simulink model "WEankle_controllerMaarten"  (R2018b)
settings: Solver=FixedStepDiscrete  StartTime=0.0  StopTime=inf  FixedStep=sampleTime  RelTol=1e-3
undefined symbols (not defined in the file or in its folder): DiscIntNeverNeededParam, forceplate, Joint_params, sampleTime
libraries: simulink x22, WE2_library x9, dspsigops x6, dspfdesign x3
(part 3 of 4)

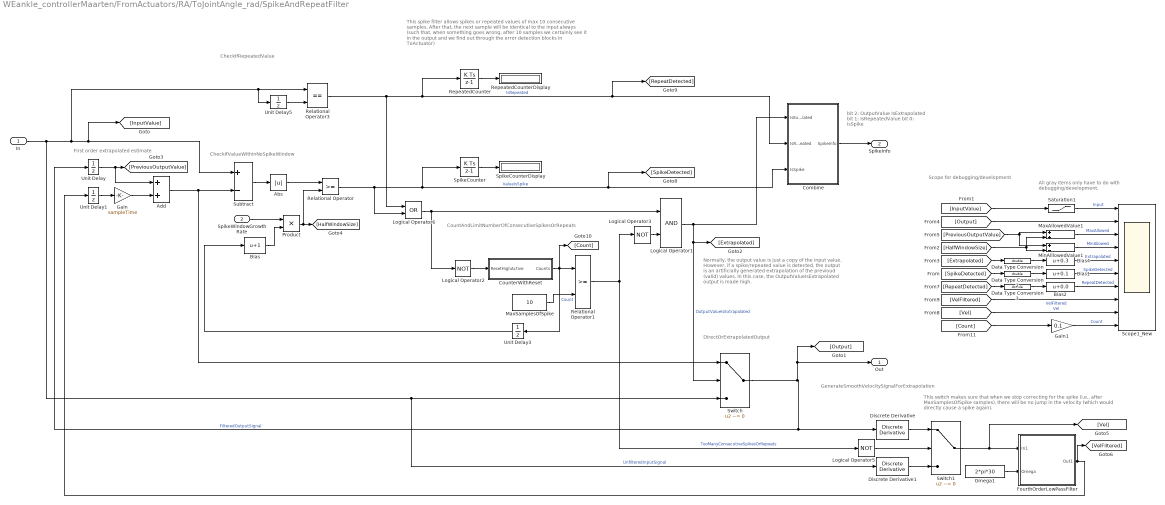
== system WEankle_controllerMaarten/FromActuators/RA/ToJointAngle_rad/SpikeAndRepeatFilter ==
  note: bit 2: OutputValue IsExtrapolated
      | bit 1: IsRepeatedValue
      | bit 0: IsSpike
  note: This switch makes sure that when we stop correcting for the spike (i.e., after MaxSamplesOfSpike samples), there will be no jump in the velocity (which would directly cause a spike again).
  note: This spike filter allows spikes or repeated values of max 10 consecutive samples. After that, the next sample will be identical to the input always (such that, when something goes wrong, after 10 samples we certainly see it in the output and we find out through the error detection blocks in ToActuator)
  note: First order extrapolated estimate
  note: CheckIfRepeatedValue
  note: CheckIfValueWithinNoSpikeWindow
  note: CountAndLimitNumberOfConsecutiveSpikesOrRepeats
  note: DirectOrExtrapolatedOutput
  note: GenerateSmoothVelocitySignalForExtrapolation
  note: All gray items only have to do with debugging/development.
  note: Scope for debugging/development
  note: Normally, the output value is just a copy of the input value. However, if a spike/repeated value is detected, the output is an artificially generated extrapolation of the previoud (valid) values. In this case, the OutputValueIsExtrapolated output is made high.
  In : Inport
  SpikeWindowGrowthRate : Inport  Port=2
  Abs : Abs
  Add : Sum
  Bias : Bias  Bias=1
  Bias1 : Bias  Bias=0.1
  Bias2 : Bias  Bias=0.0
  Bias4 : Bias  Bias=0.3
  Combine : Subsystem
  CounterWithReset : Subsystem
  Data Type Conversion : DataTypeConversion  OutDataTypeStr=double
  Data Type Conversion2 : DataTypeConversion  OutDataTypeStr=double
  Data Type Conversion3 : DataTypeConversion  OutDataTypeStr=double
  Discrete Derivative : simulink/Discrete/Discrete Derivative  gainval=1.0  ICPrevScaledInput=0.0  OutMin=[]  OutMax=[]  OutDataType=fixdt(1, 16)  OutScaling=2^-10  DoSatur=off
  Discrete Derivative1 : simulink/Discrete/Discrete Derivative  gainval=1.0  ICPrevScaledInput=0.0  OutMin=[]  OutMax=[]  OutDataType=fixdt(1, 16)  OutScaling=2^-10  DoSatur=off
  FourthOrderLowPassFilter : Subsystem
  Gain : Gain  Gain=sampleTime
  Gain1 : Gain  Gain=0.1
  Logical Operator1 : Logic  AllPortsSameDT=off  OutDataTypeStr=boolean
  Logical Operator2 : Logic  Operator=NOT  AllPortsSameDT=off  OutDataTypeStr=boolean
  Logical Operator3 : Logic  Operator=NOT  AllPortsSameDT=off  OutDataTypeStr=boolean
  Logical Operator5 : Logic  Operator=NOT  AllPortsSameDT=off  OutDataTypeStr=boolean
  Logical Operator6 : Logic  Operator=OR  AllPortsSameDT=off  OutDataTypeStr=boolean
  MaxAllowedValue1 : Sum
  MaxSamplesOfSpike : Constant  Value=10
  MinAlllowedValue1 : Sum  Inputs=+-
  Omega1 : Constant  Value=2*pi*30  OutDataTypeStr=double
  Product : Product
  Relational Operator : RelationalOperator  OutDataTypeStr=boolean  RndMeth=Nearest
  Relational Operator1 : RelationalOperator  OutDataTypeStr=boolean  RndMeth=Nearest
  Relational Operator3 : RelationalOperator  Operator===  OutDataTypeStr=boolean  RndMeth=Simplest
  RepeatedCounter : DiscreteIntegrator  SampleTime=-1  ICPrevOutput=DiscIntNeverNeededParam  ICPrevScaledInput=DiscIntNeverNeededParam
  RepeatedCounterDisplay : Display
  Saturation1 : Saturate  UpperLimit=6  LowerLimit=-6
  Scope1_New : Scope  NumInputPorts=10
  SpikeCounter : DiscreteIntegrator  SampleTime=-1  ICPrevOutput=DiscIntNeverNeededParam  ICPrevScaledInput=DiscIntNeverNeededParam
  SpikeCounterDisplay : Display
  Subtract : Sum  Inputs=+-
  Switch : Switch  Criteria=u2 ~= 0
  Switch1 : Switch  Criteria=u2 ~= 0
  Unit Delay{,1,3,5} (4 alike) : UnitDelay  SampleTime=sampleTime
  Out : Outport
  SpikeInfo : Outport  Port=2
  wires:
  Combine/1(SpikeInfo) -> SpikeInfo/1
  SpikeCounter/1 -> SpikeCounterDisplay/1
  RepeatedCounter/1 -> RepeatedCounterDisplay/1
  Logical Operator5/1 -> Switch1/2
  [Count] -> Gain1/1
  Gain1/1 -> Scope1_New/10  "Count"
  Relational Operator1/1 -> Logical Operator3/1, Logical Operator5/1  "TooManyConsecutiveSpikesOrRepeats"
  In/1 -> Discrete Derivative1/1, Switch/3, Unit Delay5/1, Relational Operator3/1, [InputValue], Subtract/1  "UnfilteredInputSignal"
  Unit Delay3/1 -> Bias/1
  Bias/1 -> Product/2
  SpikeWindowGrowthRate/1 -> Product/1
  Switch/1 -> [Output], Out/1, Unit Delay/1, Discrete Derivative/1  "FilteredOutputSignal"
  Add/1 -> Switch/1, Subtract/2
  Logical Operator1/1 -> Combine/1(IsExtrapolated), [Extrapolated], Switch/2  "OutputValueIsExtrapolated"
  Gain/1 -> Add/2
  Logical Operator6/1 -> Logical Operator1/1, Logical Operator2/1
  Unit Delay/1 -> [PreviousOutputValue], Add/1
  Abs/1 -> Relational Operator/1
  Subtract/1 -> Abs/1
  Product/1 -> Relational Operator/2, [HalfWindowSize]
  CounterWithReset/1(Counts) -> Relational Operator1/1, [Count], Unit Delay3/1  "Count"
  MaxSamplesOfSpike/1 -> Relational Operator1/2
  Discrete Derivative/1 -> Switch1/1
  Logical Operator3/1 -> Logical Operator1/2
  Discrete Derivative1/1 -> Switch1/3
  Unit Delay1/1 -> Gain/1
  Logical Operator2/1 -> CounterWithReset/1(ResetHighActive)
  Switch1/1 -> [Vel], FourthOrderLowPassFilter/1(In1)
  Omega1/1 -> FourthOrderLowPassFilter/2(Omega)
  FourthOrderLowPassFilter/1(Out1) -> [VelFiltered], Unit Delay1/1
  [Vel] -> Scope1_New/9  "Vel"
  Bias4/1 -> Scope1_New/5  "Extrapolated"
  Data Type Conversion2/1 -> Bias1/1
  [PreviousOutputValue] -> MaxAllowedValue1/1, MinAlllowedValue1/1
  [VelFiltered] -> Scope1_New/8  "VelFiltered"
  [Extrapolated] -> Data Type Conversion/1
  Data Type Conversion3/1 -> Bias2/1
  [InputValue] -> Saturation1/1
  Saturation1/1 -> Scope1_New/1  "Input"
  [SpikeDetected] -> Data Type Conversion2/1
  [Output] -> Scope1_New/2
  [RepeatDetected] -> Data Type Conversion3/1
  MaxAllowedValue1/1 -> Scope1_New/3  "MaxAllowed"
  MinAlllowedValue1/1 -> Scope1_New/4  "MinAllowed"
  [HalfWindowSize] -> MinAlllowedValue1/2, MaxAllowedValue1/2
  Data Type Conversion/1 -> Bias4/1
  Unit Delay5/1 -> Relational Operator3/2
  Relational Operator3/1 -> Logical Operator6/1, [RepeatDetected], Combine/2(IsRepeated), RepeatedCounter/1  "IsRepeated"
  Relational Operator/1 -> Logical Operator6/2, SpikeCounter/1, Combine/3(IsSpike), [SpikeDetected]  "ValueIsSpike"
  Bias2/1 -> Scope1_New/7  "RepeatDetected"
  Bias1/1 -> Scope1_New/6  "SpikeDetected"

== system WEankle_controllerMaarten/FromActuators/RA/ToJointAngle_rad/TakeDerivative ==
  note: DiscreteDerivativeOver2Samples
  note: We provide two ways of taking the derivative here:
      | dxdt = ( x(k)- x(k -1) ) / Ts
      | dxdt = ( x(k) - x(k -2) ) / (2*Ts)
      | The reason is that in TwinCAT we get a lot of jitter, which affects half of the samples. Therefore, comparing the current sample with two samples earlier may give more accurate results. this is, however, at a cost of latency.
  In1 : Inport
  Discrete Derivative : simulink/Discrete/Discrete Derivative  gainval=1.0  ICPrevScaledInput=0.0  OutMin=[]  OutMax=[]  OutDataType=fixdt(1, 16)  OutScaling=2^-10  DoSatur=off
  Manual Switch : ManualSwitch  CurrentSetting=0
  OneOverTwoSampleTime : Gain  Gain=1/(2*sampleTime)
  Subtract : Sum  Inputs=+-
  Unit Delay : UnitDelay  SampleTime=-1
  Unit Delay1 : UnitDelay  SampleTime=-1
  Out1 : Outport
  wires:
  Discrete Derivative/1 -> Manual Switch/1
  In1/1 -> Unit Delay/1, Subtract/1, Discrete Derivative/1
  Manual Switch/1 -> Out1/1
  Unit Delay/1 -> Unit Delay1/1
  Unit Delay1/1 -> Subtract/2
  Subtract/1 -> OneOverTwoSampleTime/1
  OneOverTwoSampleTime/1 -> Manual Switch/2

== system WEankle_controllerMaarten/Ankle Controller/COMverror and perturbation/TriggerPerturbation/Perturbation sync gait phase1/If Action Subsystem ==
  In1 : Inport
  Action Port : ActionPort  ActionType=then
  Out1 : Outport
  wires:
  In1/1 -> Out1/1

== system WEankle_controllerMaarten/Ankle Controller/COMverror and perturbation/TriggerPerturbation/Perturbation sync gait phase1/If Action Subsystem1 ==
  In1 : Inport
  Action Port : ActionPort  ActionType=then
  Out1 : Outport
  wires:
  In1/1 -> Out1/1

== system WEankle_controllerMaarten/FromActuators/RA/ToJointAngle_rad/SpikeAndRepeatFilter/Combine ==
  IsExtrapolated : Inport
  IsRepeated : Inport  Port=2
  IsSpike : Inport  Port=3
  Add : Sum  Inputs=+++
  Cast To Double : DataTypeConversion  OutDataTypeStr=double
  Cast To Double1 : DataTypeConversion  OutDataTypeStr=double
  Cast To Double2 : DataTypeConversion  OutDataTypeStr=double
  Gain : Gain  Gain=4
  Gain1 : Gain  Gain=2
  SpikeInfo : Outport
  wires:
  Cast To Double2/1 -> Add/3
  Cast To Double1/1 -> Gain1/1
  Cast To Double/1 -> Gain/1
  IsExtrapolated/1 -> Cast To Double/1
  IsRepeated/1 -> Cast To Double1/1
  Add/1 -> SpikeInfo/1
  Gain1/1 -> Add/2
  Gain/1 -> Add/1
  IsSpike/1 -> Cast To Double2/1

== system WEankle_controllerMaarten/FromActuators/RA/ToJointAngle_rad/SpikeAndRepeatFilter/CounterWithReset ==
  note: Stopwatch -
      | Outputs time in seconds.
      | Reset during high level of Rest pulse
  ResetHighActive : Inport
  Counter Free-Running : simulink/Sources/Counter Free-Running  NumBits=32  tsamp=-1
  Data Type Conversion : DataTypeConversion  OutDataTypeStr=double
  Latch : Subsystem
  Subtract : Sum  Inputs=+-
  Counts : Outport
  wires:
  Counter Free-Running/1 -> Latch/1(In1), Subtract/1
  Subtract/1 -> Data Type Conversion/1
  Latch/1(Out1) -> Subtract/2  "startTime"
  Data Type Conversion/1 -> Counts/1
  ResetHighActive/1 -> Latch/Enable

== system WEankle_controllerMaarten/FromActuators/RA/ToJointAngle_rad/SpikeAndRepeatFilter/FourthOrderLowPassFilter ==
  In1 : Inport
  Omega : Inport  Port=2
  Filter1 : MATLAB Function  TreatAsAtomicUnit=on  mask{sampleTime=sampleTime}
      mask prompts: sampleTime "Sample Time"
  Filter2 : MATLAB Function  TreatAsAtomicUnit=on  mask{sampleTime=sampleTime}
      mask prompts: sampleTime "Sample Time"
  Out1 : Outport
  wires:
  Omega/1 -> Filter1/2(OmegaFilter), Filter2/2(OmegaFilter)
  Filter2/1(y) -> Out1/1
  Filter1/1(y) -> Filter2/1(x)
  In1/1 -> Filter1/1(x)

== system WEankle_controllerMaarten/FromActuators/RA/ToJointAngle_rad/SpikeAndRepeatFilter/CounterWithReset/Latch ==
  In1 : Inport
  Enable : EnablePort
  Out1 : Outport
  wires:
  In1/1 -> Out1/1

== matlab function WEankle_controllerMaarten/Ankle Controller/Eventdetection/StrideTimeEstimator/MATLAB Function ==
  data: fLeftCross input; fLeftThresh input; phase_left output; fRightCross input; fRightThresh input; time input; phase_right output
function [phase_left, phase_right] = fcn(fLeftCross, fLeftThresh, fRightCross, fRightThresh, time)

persistent time_heel2heel_right
persistent time_heellast_right
persistent tdm_right
persistent time_heel2heel_left
persistent time_heellast_left
persistent tdm_left

if(isempty(time_heel2heel_left))
   time_heel2heel_right = zeros(4,1);
   time_heellast_right = -1e5;
   tdm_right = 0.1;
   
   time_heel2heel_left = zeros(4,1);
   time_heellast_left = -1e5;
   tdm_left = 0.1;
end
%% left
phase_left = (time - time_heellast_left)/(tdm_left+eps)*100;
if(fLeftCross~=0||(phase_left>100&&fLeftThresh==1))
    td_new  = time - time_heellast_left;
    if((td_new>0.8*tdm_left)||any(time_heel2heel_left>10))
        time_heellast_left = time;
        time_heel2heel_left(2:end) = time_heel2heel_left(1:end-1);
        time_heel2heel_left(1) = td_new;
        tdm_left = mean(time_heel2heel_left);
    end
end


%% right
phase_right = (time - time_heellast_right)/(tdm_right+eps)*100;
if(fRightCross~=0||(phase_right>100&&fRightThresh==1))
    td_new  = time - time_heellast_right;
    if((td_new>0.8*tdm_right)||any(time_heel2heel_right>10))
        time_heellast_right = time;
        time_heel2heel_right(2:end) = time_heel2heel_right(1:end-1);
        time_heel2heel_right(1) = td_new;
        tdm_right = mean(time_heel2heel_right);
    end
end

== matlab function WEankle_controllerMaarten/Ankle Controller/Eventdetection/COP detection (treadmill)/MATLAB Function1 ==
  data: x input; y output; OmegaFilter input; sampleTime input
function y = Filter2ndOrder(x, OmegaFilter, sampleTime)
%#codegen

persistent yd_prev y_prev;
if isempty(yd_prev)
    yd_prev = zeros(6,1); 
    y_prev = zeros(6,1);  %Derivative of the above signal
end

% Do 2nd order filtering with given omega and zeta=0.7; input of filter
% is vel_inc_sampleTime_unfilt; output is y (we assign to vel_inc_s
% later). 
if OmegaFilter==0 || isinf(OmegaFilter)
    y = x;
    y_prev = y;
    yd_prev = zeros(6,1); 
else
    zeta = 0.7;
    ydd = OmegaFilter^2 * (x - y_prev) - 2*zeta*OmegaFilter* yd_prev;
    yd = yd_prev + ydd * sampleTime;
    y = y_prev + yd * sampleTime;

    y_prev = y; yd_prev = yd;
end

== matlab function WEankle_controllerMaarten/Ankle Controller/MATLAB Function5 ==
  data: e0 input; G input; SolGains output; COMd input
function SolGains  = CombineSoleusGains(e0,G,COMd)
% input arguments:

SolGains = [e0; G; COMd];

== matlab function WEankle_controllerMaarten/ForcePlate/Calibration/MATLAB Function ==
  data: left input; left_calib output; right input; start input; right_calib output; caltime_s input
function [left_calib, right_calib] = calibrateOffset(left, right, start, caltime_s)
persistent calibrated
persistent offcum_left
persistent offcum_right
persistent counter
persistent nosamp

if(isempty(calibrated))
   calibrated = false;
   offcum_left = left*0;
   offcum_right = right*0;
   counter = 0;
   nosamp = max(1, floor(caltime_s*1000));
end

if(start == 1)
    counter = 0;
    calibrated = false;
    offcum_left = left*0;
    offcum_right = right*0;
    nosamp = max(1, floor(caltime_s*1000));
end

if(calibrated)
    left_calib = left - offcum_left;
    right_calib = right - offcum_right;
else
    if(~calibrated)
        counter = counter + 1;
        offcum_left = offcum_left + left/(nosamp);
        offcum_right = offcum_right + right/(nosamp);
        if(counter >= nosamp)
            calibrated = true;
        end
    end
    left_calib = left;
    right_calib = right;
end

== matlab function WEankle_controllerMaarten/Ankle Controller/Eventdetection/COP detection (treadmill)/MATLAB Function2 ==
  data: x input; y output; OmegaFilter input; sampleTime input
function y = Filter2ndOrder(x, OmegaFilter, sampleTime)
%#codegen

persistent yd_prev y_prev;
if isempty(yd_prev)
    yd_prev = zeros(6,1); 
    y_prev = zeros(6,1);  %Derivative of the above signal
end

% Do 2nd order filtering with given omega and zeta=0.7; input of filter
% is vel_inc_sampleTime_unfilt; output is y (we assign to vel_inc_s
% later). 
if OmegaFilter==0 || isinf(OmegaFilter)
    y = x;
    y_prev = y;
    yd_prev = zeros(6,1); 
else
    zeta = 0.7;
    ydd = OmegaFilter^2 * (x - y_prev) - 2*zeta*OmegaFilter* yd_prev;
    yd = yd_prev + ydd * sampleTime;
    y = y_prev + yd * sampleTime;

    y_prev = y; yd_prev = yd;
end

== matlab function WEankle_controllerMaarten/Ankle Controller/COMverror and perturbation/TriggerPerturbation/Perturbation sync gait phase1/TimeBetweenPert ==
  data: TimeBetweenPert input; timesvector input; Allow output; Delivered input
function Allow = fcn(TimeBetweenPert,timesvector,Delivered)
% To randomize the time between perturbations (min 6s)
persistent i 
persistent TimeSelector 
persistent flagfirst %flag to indicate first time
if isempty(i)
    i = 1;
    flagfirst = 1;
end
if Delivered == 1 && ~flagfirst %Perturbation delivered. Go to next element of timesVector avoiding a false entrance the first time
    i = i+1;
end
%% Assign new time
len = length(timesvector);
if i > len %reset the index when all perturbations from the vector are done
    i = 1;
end
TimeSelector = timesvector(i);

if TimeSelector < 6
    TimeSelector = 6;
end
%% Allow new perturbation or not
if TimeBetweenPert >= TimeSelector
    Allow = 1;
else
    Allow = 0;
end
%%
flagfirst = 0;

== matlab function WEankle_controllerMaarten/Ankle Controller/Eventdetection/Subsystem/MATLAB Function ==
  data: f input; y output; nf input; nf_1 input; th input
function y = fcn(f,nf,nf_1,th)

maxCounter = 200; %time to wait in zero
persistent counter
persistent out
if isempty(counter)
    counter = maxCounter+1;
    out = f;
end

if (nf == 0) && (nf_1 < -50)
    out = 0;
    counter = 0;
else
    counter = counter+1;
    if counter > maxCounter
        if (f > -th) && (f < th) && (nf == 0)
            out = 0;
        else
            out = f;
        end
    end
end

y = out;

== matlab function WEankle_controllerMaarten/Ankle Controller/Eventdetection/StrideTimeEstimator/MATLAB Function3 ==
  data: fLeftCross input; fLeftThresh input; phase_left output; fRightCross input; fRightThresh input; time input; phase_right output; SingleL input; SingleR input; reset input
function [phase_left, phase_right] = fcn(fLeftCross, fLeftThresh, fRightCross, fRightThresh, time, SingleL, SingleR, reset)

persistent time_heel2heel_right
persistent time_heellast_right
persistent tdm_right
persistent time_heel2heel_left
persistent time_heellast_left
persistent tdm_left
persistent  phase_left2
persistent  phase_right2

if(isempty(time_heel2heel_left) || reset==1)
   time_heel2heel_right = zeros(4,1);
   time_heellast_right = -1e5;
   tdm_right = 0.1;
   
   time_heel2heel_left = zeros(4,1);
   time_heellast_left = -1e5;
   tdm_left = 0.1;
   
    phase_left2 = 0; %Used to reset the left phase when prepositioning of left leg is detected (SingleL 1 to 0)
    phase_right2 = 0; %Used to reset the right phase when prepositioning of right leg is detected (SingleR 1 to 0)
end
%% left
phase_left = (time - time_heellast_left)/(tdm_left+eps)*100 - phase_left2;
% if(fLeftCross~=0||(phase_left>100&&fLeftThresh==1))

if(SingleR)
    phase_left2 = phase_left;
end
if((fLeftCross~=0||(phase_left>100&&fLeftThresh==1)))
    td_new  = time - time_heellast_left;
    phase_left2 = 0;
    if((td_new>0.8*tdm_left)||any(time_heel2heel_left>10))
        time_heellast_left = time;
        time_heel2heel_left(2:end) = time_heel2heel_left(1:end-1);
        time_heel2heel_left(1) = td_new;
        tdm_left = mean(time_heel2heel_left);
    end
end


%% right
phase_right = (time - time_heellast_right)/(tdm_right+eps)*100 - phase_right2;
% if(fRightCross~=0||(phase_right>100&&fRightThresh==1))
if(SingleL)
    phase_right2 = phase_right;
end
if(fRightCross~=0||(phase_right>100&&fRightThresh==1))
    td_new  = time - time_heellast_right;
    phase_right2 = 0;
    if((td_new>0.8*tdm_right)||any(time_heel2heel_right>10))
        time_heellast_right = time;
        time_heel2heel_right(2:end) = time_heel2heel_right(1:end-1);
        time_heel2heel_right(1) = td_new;
        tdm_right = mean(time_heel2heel_right);
    end
end

== matlab function WEankle_controllerMaarten/FromActuators/RA/CheckOperationEnabled ==
  data: u input; y output
function y = fcn(u)
%#codegen
% Extract the 'Operation Enabled' bit from the Status Word
y = double(bitget(u, 2+1)); % bitget is one-based

== matlab function WEankle_controllerMaarten/FromActuators/RA/ToJointAngle_rad/FilterFourthOrder/Filter1 ==
  data: x input; OmegaFilter input; y output; sampleTime parameter
function y = Filter2ndOrder(x, OmegaFilter, sampleTime)
%#codegen

persistent yd_prev y_prev;
if isempty(yd_prev)
    yd_prev = 0; 
    y_prev = 0; %Derivative of the above signal
end;

% Do 2nd order filtering with given omega and zeta=0.7; input of filter
% is vel_inc_sampleTime_unfilt; output is y (we assign to vel_inc_s
% later). 
if OmegaFilter==0 || isinf(OmegaFilter)
    y=x;
    y_prev=y;
    yd_prev =0;
else
    zeta = 0.7;
    ydd = OmegaFilter^2 * (x - y_prev) - 2*zeta*OmegaFilter* yd_prev;
    yd = yd_prev + ydd * sampleTime;
    y = y_prev + yd * sampleTime;

    y_prev = y; yd_prev = yd;
end;

== matlab function WEankle_controllerMaarten/Ankle Controller/Eventdetection/Heels movement/MATLAB Function2 ==
  data: gainL output; COPyL input; gainR output; COPyR input
function [gainL,gainR] = Stance(COPyL,COPyR)
%#codegen
if COPyR == 0
    gainR = 0;
else
    gainR = 1;
end

if COPyL == 0
    gainL = 0;
else
    gainL = 1;
end

end

== matlab function WEankle_controllerMaarten/Ankle Controller/COMverror and perturbation/TriggerPerturbation/PushOrPull ==
  data: Perturb input; vectorPushPull input; NewPert output; Delivered input
function NewPert = fcn(Perturb,vectorPushPull,Delivered)
% To randomize pushes and pulls
persistent i 
persistent Selector 
persistent flagfirst %flag to indicate first time
if isempty(i)
    i = 1;
    flagfirst = 1;
end
if Delivered == 1 && ~flagfirst %Perturbation delivered. Go to next element of timesVector avoiding a false entrance the first time
    i = i+1;
end
%%
len = length(vectorPushPull);
if i > len %reset the index when all perturbations from the vector are done
    i = 1;
end
Selector = vectorPushPull(i);

if Selector < -1
    Selector = -1;
elseif Selector > 1
    Selector = 1;
end
%% 
NewPert = Selector*Perturb;
%%
flagfirst = 0;

== matlab function WEankle_controllerMaarten/Ankle Controller/COMverror and perturbation/COMvError/MATLAB Function1 ==
  data: ShutDown input; PertDetect input; TriggerPush output
function TriggerPush = fcn(ShutDown,PertDetect)
if ShutDown == 0
    TriggerPush = PertDetect;
else
    TriggerPush = 0;
end

== matlab function WEankle_controllerMaarten/Ankle Controller/COMverror and perturbation/COMvError/Signal learner/MATLAB Function ==
  data: reset input; t input; trigger input; signal input; signal_learned output; n_strides_ output; n_ output; m_ output; output_duration_ output; n_rep input; perturbation output; threshPert input; DataLost input; ShutDown output
function [signal_learned,n_strides_,n_,m_,output_duration_,perturbation,ShutDown] = signal_learner(reset,t,trigger,signal,n_rep,threshPert,DataLost)
%     n_rep = how many signals period will be averaged
n_storage = 2000; %stored signal will be 2000 elements long. playback will be interpolated
n_buffer_size = 4000; %can maximally read 4000;
perturbation = 0;
ShutDown = 0; %No trigger the controller if DataLost or if we are in the first n_rep strides
persistent n %elements of vector
persistent n_strides % total number of strides
persistent m %Pointer for recording each stride in buffer (1:n_rep)
persistent t0 % moment in time of last stride
persistent last_buffer
persistent output_signal_buffer
persistent output_signal
persistent output_duration
persistent output_duration_buffer
persistent maximums
persistent MaxAver

if isempty(n)
    n = 1;
    m = 1;
    t0 = 0;
    last_buffer = zeros(1,n_buffer_size);
    output_signal_buffer = zeros(n_rep,n_storage);
    output_signal = zeros(1,n_storage);
    output_duration_buffer = zeros(n_rep,1);
    n_strides = 0;
    output_duration = 1;
    % Added Cristina
    maximums = 200*ones(n_rep,1); %to store the maximums of previous steps
    MaxAver = 200; % This number multiplied by 1.5 is the one above which a perturbation is supposed to happen,
    %     and thereby, that step will be excluded to calculate the mean
end
if ~DataLost && ~reset
    t_rel = t-t0;
    if (trigger && t_rel > 0.1) %if trigger happens, note down the absolute time when that was
        n_strides = n_strides+1; %counting number of strides
        last_stride_duration = t-t0;
        
        t0 = t; %Reset the moment when the last stride happened
        %% Added Cristina
        % See if there was a perturbation in the last step
        Perturbation = 0; % Init perturbation in the last step
        leng = length(last_buffer(1:min([n,n_buffer_size])));
        for i = 1:leng
            element = last_buffer(i);
            if element > 1.5*MaxAver % A perturbation was detected in the last step
                Perturbation = 1;
            end
        end
        
        %% Changed Cristina
        if n_strides >= 3
            if (last_stride_duration > 0.5*output_duration)% to avoid false triggers
                enter = 1;
            else
                enter = 0;
            end
        else
            enter = 1;
        end
        if (last_stride_duration > 0) && enter % otherwise failure at start or false trigger  
            % If there was no perturbation, take that step into account.
            % Otherwise, exclude it
            if ~Perturbation %in the last step
                %interpolate regardless of last duration to n_storage elements
%                 if n == 1
%                     n = n+1;
%                 end
                output_signal_buffer(m,:) = ...
                    interp1(...
                    linspace(0,last_stride_duration,n),... %vector of n elements
                    last_buffer(1:min([n,n_buffer_size])),... %only read up to incl. n elements, if bigger than n_buffer size, then we need to limit.
                    linspace(0,last_stride_duration,n_storage)); %remap that to a new 'x' with n_storage elements
                output_signal = mean(output_signal_buffer); %averages over n_rep stored signals
                
                output_duration_buffer(m) = last_stride_duration;
                output_duration = mean(output_duration_buffer); %duration is average of last n_rep times
                
                maximums(m) = max(last_buffer(1:min([n,n_buffer_size]))); %store the new maximum of current step
                MaxAver = mean(maximums); %calculate the average of maximums found in the last n_rep
                
                m = m+1;
                if m > n_rep
                    m = 1;
                end
            end
            if (n_strides <= n_rep)
                output_duration = last_stride_duration;
            end
            %last_buffer = zeros() %is not required due to 1:n
            n = 1;
        end
    end
end
if ~DataLost && ~reset
    %% process input
    t_rel = t-t0;
    last_buffer(min([n n_buffer_size])) = signal;
    
    %% generate output
    fractional_index = t_rel/output_duration * (n_storage-1);
    rounded_index = min([1+floor(fractional_index),n_storage]); %cannot overflow
    fraction = 1+fractional_index - rounded_index;
    
    %linearly interpolate
    if (rounded_index >= n_storage - 1)
        signal_learned = output_signal(n_storage-1);
    else
        signal_learned = output_signal(rounded_index)*(1-fraction) + output_signal(rounded_index+1)*fraction;
    end
    
    %debug output
    n_strides_ = n_strides;
    n_ = n;
    m_ = m;
    output_duration_ = output_duration;
    if signal > threshPert*MaxAver
        perturbation = 1;
    end
else
    %debug output
    n_strides_ = n_strides;
    n_ = n;
    m_ = m;
    output_duration_ = output_duration;
    perturbation = 0;
    signal_learned = 0;
end

%do not output anything learned in first n_rep strides.
if (n_strides <= n_rep) || DataLost || reset
    signal_learned = 0;
    output_duration_ = 0;%last_stride_duration;
    ShutDown = 1;
end
if ~DataLost && ~reset
    %shift signal storage pointer, avoid overflow
    n = n+1;
else
    n = 1;
end
end

== matlab function WEankle_controllerMaarten/Ankle Controller/COMverror and perturbation/COMvError/Data lost detection/MATLAB Function1 ==
  data: u input; y output; u_1 input
function y = fcn(u,u_1)
% input signal u = xVelCOM
% output y = data lost detection (1 or 0)
y = 0;
if u == u_1 % The new data is equal to the previous one --> See how Qualisys will send it since NaN is not supported
    y = 1; % Data lost
else
    y = 0; % Data good
end

== matlab function WEankle_controllerMaarten/Ankle Controller/COMverror and perturbation/COMvError/Data lost detection/MATLAB Function2 ==
  data: DataLost input; DataLost_1 input; ErrorOut output; ErrorIn input; avoid output
function [ErrorOut,avoid] = fcn(DataLost,DataLost_1,ErrorIn)
% ErrorOut is the new error corrected when data lost

maxCounter = 1500; %time to wait after a DataLost detection to let the controller works again (1.5s)
persistent counter
if isempty(counter)
    counter = maxCounter+1;
end

ErrorOut = ErrorIn;
avoid = 0;

if DataLost == 1 % Data lost
    ErrorOut = 0; 
    avoid = 1;
elseif DataLost == 0 && DataLost_1 == 1 % Data just recovered after a loss
    counter = 1;
    ErrorOut = 0; 
    avoid = 1;
elseif DataLost == 0 && DataLost_1 ~= 1 % Good data
    if counter <= maxCounter % Wait 1.5s after data has been recovered to generate the newError
        ErrorOut = 0;
        avoid = 1;
        counter = counter + 1;
    else
        ErrorOut = ErrorIn;
        avoid = 0;
    end
end

== matlab function WEankle_controllerMaarten/Ankle Controller/COMverror and perturbation/COMvError/PerturbationDetectionFromError ==
  data: t input; trigger input; signal input; n_rep input; push output; maxAver output; rangeAver output; threshPert input; DataLost input
function [push,maxAver,rangeAver] = PerturbationDetectionFromError(t,trigger,signal,n_rep,threshPert,DataLost)
    n_buffer_size = 4000; %can maximally read 4000;
    push = 0; 
    
    persistent n %elements of vector
    persistent n_strides % total number of strides
    persistent m %Pointer for recording each stride in buffer (1:n_rep)
    persistent t0 % moment in time of last stride
    persistent last_buffer
    persistent maximums
    persistent MaxAver
    persistent minimums
    persistent MinAver
    persistent RangeAver

    if isempty(n)
       n = 1;
       m = 1;
       t0 = 0;
       last_buffer = zeros(1,n_buffer_size);
       n_strides = 0;

       maximums = 50*ones(n_rep,1); %to store the maximums of previous steps
       MaxAver = 50; % This number multiply by 1.5 is the one above which a push perturbation is supposed to happen,
%     and thereby, that step will be excluded to calculate the mean of
%     maximums
       minimums =  -120*ones(n_rep,1);
       MinAver = -120;
       RangeAver = 170;
    end
if ~DataLost
    t_rel = t-t0;
    if (trigger && t_rel > 0.1) %if trigger happens, note down the absolute time when that was
        n_strides = n_strides+1; %counting number of strides
        last_stride_duration = t-t0;

        t0 = t; %Reset the moment when the last stride happened
        %% Added Cristina
        % See if there was a perturbation in the last step
        Push = 0; % Init perturbation in the last step
        leng = length(last_buffer(1:min([n,n_buffer_size])));
        for i = 1:leng
            element = last_buffer(i);
            if element > 1.5*MaxAver % A perturbation was detected in the last step
                Push = 1;
            end
        end
        
        %% Changed Cristina
        if (last_stride_duration > 0) %otherwise failure at start
            % If there was no perturbation, take that step into account.
            % Otherwise, exclude it
            if ~Push %in the last step                
                maximums(m) = max(last_buffer(1:min([n,n_buffer_size]))); %store the new maximum of current step
                MaxAver = mean(maximums); %calculate the average of maximums found in the last n_rep
                
                minimums(m) = min(last_buffer(1:min([n,n_buffer_size]))); %store the new minimum of current step
                MinAver = mean(minimums); %calculate the average of minimums found in the last n_rep
                RangeAver = MaxAver - MinAver;
                
                m = m+1;
                if m > n_rep 
                    m = 1;
                end
            end

            n = 1;
        end
    end
end
if ~DataLost
    %% process new data
    last_buffer(min([n n_buffer_size])) = signal;
    
    %% generate output
    if signal > threshPert*RangeAver 
        push = 1;
    end
    maxAver = MaxAver;
    rangeAver = RangeAver;
    
else
    maxAver = MaxAver;
    rangeAver = RangeAver;
    push = 0;
end
%do not output anything learned in first n_rep strides.
if (n_strides <= n_rep) || DataLost
    push = 0;
end

if ~DataLost
    %shift signal storage pointer, avoid overflow
    n = n+1;
else
    n = 1;
end
end

== matlab function WEankle_controllerMaarten/Ankle Controller/COMverror and perturbation/COMvError/PertDetection/MATLAB Function1 ==
  data: PertFromError input; PertDetect output; PertFromInput input; avoid input; StartPertFromError input
function PertDetect = NotTriggerIfDataLost(PertFromError,PertFromInput,avoid,StartPertFromError)
% PertFromError is already including the data lost because the error will
% be zero if that happens. But it could be that PertFromInput says there is
% a perturbation, and that is why this is needed

%avoid because data lost

persistent CounterPertError
if isempty(CounterPertError)
    CounterPertError = 0;
end
if StartPertFromError
    CounterPertError = CounterPertError +1;
end
%Discard the first two perturbations detected from error
if (PertFromError || PertFromInput) && ~avoid && (CounterPertError > 2)  %Detect a new perturbation
    PertDetect = 1;
else
    PertDetect = 0;
end

== matlab function WEankle_controllerMaarten/Ankle Controller/COMverror and perturbation/COMvError/PertDetection/MATLAB Function2 ==
  data: Pert input; PertDetect output; Pert_1 input
function PertDetect = WaitForNewDetect(Pert,Pert_1)
PertDetect = 0;
% Wait 2s to trigger a new perturbation if a previous one was detected

maxCounter = 2000; %time to wait after a Perturbation detection to detect a new one
persistent counter
if isempty(counter)
    counter = maxCounter+1;
end

if Pert_1 == 0 && Pert == 1 %New possible perturbation
    if counter > maxCounter
        PertDetect = Pert;
    else
        PertDetect = 0;
    end
elseif Pert_1 == 1 && Pert == 1 %middle of a perturbation
    if counter > maxCounter
        PertDetect = Pert;
    else
        PertDetect = 0;
    end
elseif Pert_1 == 1 && Pert == 0 % end of a perturbation
    counter = 1;
    PertDetect = Pert;
end

counter = counter + 1;

== matlab function WEankle_controllerMaarten/Ankle Controller/Eventdetection/Subsystem1/MATLAB Function ==
  data: f input; y output; nf input; nf_1 input; th input
function y = fcn(f,nf,nf_1,th)

maxCounter = 200; %time to wait in zero
persistent counter
persistent out
if isempty(counter)
    counter = maxCounter+1;
    out = f;
end

if (nf == 0) && (nf_1 < -50)
    out = 0;
    counter = 0;
else
    counter = counter+1;
    if counter > maxCounter
        if (f > -th) && (f < th) && (nf == 0)
            out = 0;
        else
            out = f;
        end
    end
end

y = out;

== matlab function WEankle_controllerMaarten/Ankle Controller/Eventdetection/MATLAB Function2 ==
  data: COPyL input; leftFront output; COPyR input; rightFront output; singleLeft output; singleRight output; COPyL_1 input; COPyR_1 input
% function [LeftFront,RightFront,SingleLeft,SingleRight] = DetectionFrontFoot(COPyL,COPyR,COPyL_1,COPyR_1)
function [leftFront,rightFront,singleLeft,singleRight] = DetectionFrontFoot(COPyL,COPyR,COPyL_1,COPyR_1)
%#codegen
% LeftFront = 0; 
% RightFront = 0;
% SingleRight = 0;
% SingleLeft = 0;

persistent LeftFront
persistent RightFront
persistent SingleRight
persistent SingleLeft

maxCounter = 3; %time to wait to avoid false detection
maxCounterStance = 4;
persistent counter
persistent counterStance
if isempty(counter)
    counter = maxCounter+1;
    counterStance = maxCounterStance+1;
    LeftFront = 0;
    RightFront = 0;
    SingleRight = 0;
    SingleLeft = 0;
end

%%
if (COPyL~=0) && (COPyR~=0) && ((COPyL_1 == 0) || (COPyR_1 == 0)) %Possible init of double stance
    counterStance = 0;
elseif (COPyL~=0) && (COPyR~=0) && (COPyL_1 ~= 0) && (COPyR_1 ~= 0) % Possible double stance
    counterStance = counterStance + 1;
    if counterStance > maxCounterStance
        if COPyL > COPyR %Left in front
            LeftFront = 1;
            RightFront = 0;
            SingleRight = 0;
            SingleLeft = 0;
        elseif COPyL < COPyR %Rigth in front
            LeftFront = 0;
            RightFront = 1;
            SingleRight = 0;
            SingleLeft = 0;
        end
    end
    
% if (COPyL~=0) && (COPyR~=0) %Double stance
%     if COPyL > COPyR %Left in front
%         LeftFront = 1;
%         RightFront = 0;
%         SingleRight = 0;
%         SingleLeft = 0;
%     elseif COPyL < COPyR %Rigth in front
%         LeftFront = 0;
%         RightFront = 1;
%         SingleRight = 0;
%         SingleLeft = 0;
%     end
elseif (COPyL == 0) && (COPyR == 0) %No one on the treadmill
    LeftFront = 0;
    RightFront = 0;
    SingleRight = 0;
    SingleLeft = 0;
elseif (COPyL == 0) && (COPyL_1 ~= 0) && (COPyR ~= 0) %Init of a possible Left swing, Rigth stance
    counter = 0;
    LeftFront = 0;
    RightFront = 1;
elseif (COPyL == 0) && (COPyL_1 == 0) && (COPyR ~= 0) % Possible Left swing, Rigth stance
    counter = counter+1;
    LeftFront = 0;
    RightFront = 1;
    if counter > maxCounter
        SingleRight = 1;
        SingleLeft = 0;
    end
elseif (COPyR == 0) && (COPyR_1 ~= 0) && (COPyL ~= 0) %Init of a possible Right swing, Left stance
    counter = 0;
    LeftFront = 1;
    RightFront = 0;
elseif (COPyR == 0) && (COPyR_1 == 0) && (COPyL ~= 0) %Possible Right swing, Left stance
    counter = counter+1;
    LeftFront = 1;
    RightFront = 0;
    if counter > maxCounter
        SingleRight = 0;
        SingleLeft = 1;
    end
end

leftFront = LeftFront;
rightFront =RightFront; 
singleRight = SingleRight;
singleLeft = SingleLeft;
end

== matlab function WEankle_controllerMaarten/Ankle Controller/MATLAB Function6 ==
  data: e0 input; G input; loff input; GSol input; TibGains output; COMd input
function TibGains  = CombineTibGains(e0,G,loff,GSol,COMd)
% input arguments:

TibGains = [e0; G; loff; GSol; COMd];

== matlab function WEankle_controllerMaarten/Ankle Controller/COMverror and perturbation/TriggerPerturbation/MATLAB Function2 ==
  data: Trigger output; SingleR input; SingleL input; PhaseL input; PhaseR input; GRFzL input; TypePert input; Delivered input
function Trigger   = Trigger(SingleR, SingleL, PhaseL, PhaseR, GRFzL, TypePert, Delivered)
%#codegen
% TypePert is vector with perturbations type 1-(Double stance rigth front) or 2-(middle left swing)
persistent i % index to go through TypePert vector
persistent delivered
persistent flagfirst %flag to indicate first time
if isempty(i)
    i = 1;
    flagfirst = 1;
end
delivered = Delivered;
if delivered == 1 && ~flagfirst %Perturbation delivered. Go to next element of TypePert avoiding a false entrance the first time
    i = i+1;
    delivered = 0; % not sure if neccessary 
end

len = length(TypePert);
if i > len %reset the index when all perturbations from the vector are done
    i = 1;
end
Pert = TypePert(i);

%%
Trigger = 0;
%% Left swing
% Left swing phase (SingleR == 1) -- Torque to right foot
if SingleR == 1
    % Start left swing %TypePert=1
%     if ((10 <= PhaseR) && (PhaseR < 20)) && (Pert == 1)
%         Trigger = 1; 
    % Middle left swing %TypePert=2
%     elseif ((GRFzL < 30) && (20 <= PhaseR) && (PhaseR < 40)) && (Pert == 2)
    if ((GRFzL < 30) && (20 <= PhaseR) && (PhaseR < 40) && (70 <= PhaseL) && (PhaseL < 90)) && (Pert == 2)
        Trigger = 1;
    else
        Trigger = 0;
    end
end

%% Double stance (SingleR == 0 && SingleL == 0) -- Torques to both feet
if ((SingleR == 0) && (SingleL == 0))
   % Right in front - beginning of double stance %TypePert=1
   if ((0 <= PhaseR) && (PhaseR < 7) && (49 <= PhaseL) && (PhaseL < 60)) && (Pert == 1)
       Trigger = 1;
%    % Left in front - beginning of double stance
%    elseif ((50 < PhaseR) && (PhaseR < 70))
%        Trigger = 1;
   else
       Trigger = 0;
   end
end
flagfirst = 0;

== matlab function WEankle_controllerMaarten/FromActuators/RA/ToJointAngle_rad/FilterFourthOrder/Filter2 ==
  data: x input; OmegaFilter input; y output; sampleTime parameter
function y = Filter2ndOrder(x, OmegaFilter, sampleTime)
%#codegen

persistent yd_prev y_prev;
if isempty(yd_prev)
    yd_prev = 0; 
    y_prev = 0; %Derivative of the above signal
end;

% Do 2nd order filtering with given omega and zeta=0.7; input of filter
% is vel_inc_sampleTime_unfilt; output is y (we assign to vel_inc_s
% later). 
if OmegaFilter==0 || isinf(OmegaFilter)
    y=x;
    y_prev=y;
    yd_prev =0;
else
    zeta = 0.7;
    ydd = OmegaFilter^2 * (x - y_prev) - 2*zeta*OmegaFilter* yd_prev;
    yd = yd_prev + ydd * sampleTime;
    y = y_prev + yd * sampleTime;

    y_prev = y; yd_prev = yd;
end;

== matlab function WEankle_controllerMaarten/FromActuators/RA/ToJointAngle_rad/MATLAB Function ==
  data: u input; y output int32; counts_rev input; dowrap input
function y = wrapAroundZero(u, counts_rev, dowrap)
%#codegen
%
% Depending on the value of dowrap, this function does the following:
% dowrap == 0 -> pass u unchanged; i.e., y=u; (normal case)
%                This implies that at u=0 a 'jump' of one full turn is
%                seen. If 0 is not within the range of motion, this is
%                acceptable (you always have a jump somewhere).
% dowrap == 1 -> Interpret u as a couts_rev-size _signed_ integer, and output 
%                the value of this signed integer as y. In this case, the
%                'jump' is at counts_rev/2. Use this case when 0 is within
%                the range of motion (and counts_rev/2 is outside it).
% Since the range of motion of each joint is less than pi, there is always
% one of the above possibilities that can be chosen (in other words, there
% is always at least one of [0, counts_rev/2] outside the range of motion).
%                
if ~dowrap
    y = int32(u); % The counts_rev is in our case 2^20, so this gives no danger of being outside the range of an int32.
                  % (note that u is a uint32)
else
    % Do the wrapping
    if u <= abs(counts_rev)/2
        y=int32(u);
    else
        y=int32(u) - int32(abs(counts_rev));
    end;
end;

== matlab function WEankle_controllerMaarten/FromActuators/RA/ToJointAngle_rad/MATLAB Function1 ==
  data: u input; y output int32; counts_rev input; dowrap input
function y = wrapAroundZero(u, counts_rev, dowrap)
%#codegen
%
% Depending on the value of dowrap, this function does the following:
% dowrap == 0 -> pass u unchanged; i.e., y=u; (normal case)
%                This implies that at u=0 a 'jump' of one full turn is
%                seen. If 0 is not within the range of motion, this is
%                acceptable (you always have a jump somewhere).
% dowrap == 1 -> Interpret u as a couts_rev-size _signed_ integer, and output 
%                the value of this signed integer as y. In this case, the
%                'jump' is at counts_rev/2. Use this case when 0 is within
%                the range of motion (and counts_rev/2 is outside it).
% Since the range of motion of each joint is less than pi, there is always
% one of the above possibilities that can be chosen (in other words, there
% is always at least one of [0, counts_rev/2] outside the range of motion).
%                
if ~dowrap
    y = int32(u); % The counts_rev is in our case 2^20, so this gives no danger of being outside the range of an int32.
                  % (note that u is a uint32)
else
    % Do the wrapping
    if u <= abs(counts_rev)/2
        y=int32(u);
    else
        y=int32(u) - int32(abs(counts_rev));
    end;
end;

== matlab function WEankle_controllerMaarten/FromActuators/RA/ToJointAngle_rad/SpikeAndRepeatFilter/FourthOrderLowPassFilter/Filter1 ==
  data: x input; OmegaFilter input; y output; sampleTime parameter
function y = Filter2ndOrder(x, OmegaFilter, sampleTime)
%#codegen

persistent yd_prev y_prev;
if isempty(yd_prev)
    yd_prev = 0; 
    y_prev = 0; %Derivative of the above signal
end;

% Do 2nd order filtering with given omega and zeta=0.7; input of filter
% is vel_inc_sampleTime_unfilt; output is y (we assign to vel_inc_s
% later). 
if OmegaFilter==0 || isinf(OmegaFilter)
    y=x;
    y_prev=y;
    yd_prev =0;
else
    zeta = 0.7;
    ydd = OmegaFilter^2 * (x - y_prev) - 2*zeta*OmegaFilter* yd_prev;
    yd = yd_prev + ydd * sampleTime;
    y = y_prev + yd * sampleTime;

    y_prev = y; yd_prev = yd;
end;

== matlab function WEankle_controllerMaarten/FromActuators/RA/ToJointAngle_rad/SpikeAndRepeatFilter/FourthOrderLowPassFilter/Filter2 ==
  data: x input; OmegaFilter input; y output; sampleTime parameter
function y = Filter2ndOrder(x, OmegaFilter, sampleTime)
%#codegen

persistent yd_prev y_prev;
if isempty(yd_prev)
    yd_prev = 0; 
    y_prev = 0; %Derivative of the above signal
end;

% Do 2nd order filtering with given omega and zeta=0.7; input of filter
% is vel_inc_sampleTime_unfilt; output is y (we assign to vel_inc_s
% later). 
if OmegaFilter==0 || isinf(OmegaFilter)
    y=x;
    y_prev=y;
    yd_prev =0;
else
    zeta = 0.7;
    ydd = OmegaFilter^2 * (x - y_prev) - 2*zeta*OmegaFilter* yd_prev;
    yd = yd_prev + ydd * sampleTime;
    y = y_prev + yd * sampleTime;

    y_prev = y; yd_prev = yd;
end;

== matlab function WEankle_controllerMaarten/FromActuators/RA/ToJointTorque/MATLAB Function ==
  data: u input; y output int32; counts_rev input; dowrap input
function y = wrapAroundZero(u, counts_rev, dowrap)
%#codegen
%
% Depending on the value of dowrap, this function does the following:
% dowrap == 0 -> pass u unchanged; i.e., y=u; (normal case)
%                This implies that at u=0 a 'jump' of one full turn is
%                seen. If 0 is not within the range of motion, this is
%                acceptable (you always have a jump somewhere).
% dowrap == 1 -> Interpret u as a couts_rev-size _signed_ integer, and output 
%                the value of this signed integer as y. In this case, the
%                'jump' is at counts_rev/2. Use this case when 0 is within
%                the range of motion (and counts_rev/2 is outside it).
% Since the range of motion of each joint is less than pi, there is always
% one of the above possibilities that can be chosen (in other words, there
% is always at least one of [0, counts_rev/2] outside the range of motion).
%                
if ~dowrap
    y = int32(u); % The counts_rev is in our case 2^20, so this gives no danger of being outside the range of an int32.
                  % (note that u is a uint32)
else
    % Do the wrapping
    if u <= abs(counts_rev)/2
        y=int32(u);
    else
        y=int32(u) - int32(abs(counts_rev));
    end;
end;

== matlab function WEankle_controllerMaarten/FromActuators/RA/ToJointTorque/MATLAB Function1 ==
  data: u input; y output int32; counts_rev input; dowrap input
function y = wrapAroundZero(u, counts_rev, dowrap)
%#codegen
%
% Depending on the value of dowrap, this function does the following:
% dowrap == 0 -> pass u unchanged; i.e., y=u; (normal case)
%                This implies that at u=0 a 'jump' of one full turn is
%                seen. If 0 is not within the range of motion, this is
%                acceptable (you always have a jump somewhere).
% dowrap == 1 -> Interpret u as a couts_rev-size _signed_ integer, and output 
%                the value of this signed integer as y. In this case, the
%                'jump' is at counts_rev/2. Use this case when 0 is within
%                the range of motion (and counts_rev/2 is outside it).
% Since the range of motion of each joint is less than pi, there is always
% one of the above possibilities that can be chosen (in other words, there
% is always at least one of [0, counts_rev/2] outside the range of motion).
%                
if ~dowrap
    y = int32(u); % The counts_rev is in our case 2^20, so this gives no danger of being outside the range of an int32.
                  % (note that u is a uint32)
else
    % Do the wrapping
    if u <= abs(counts_rev)/2
        y=int32(u);
    else
        y=int32(u) - int32(abs(counts_rev));
    end;
end;

== matlab function WEankle_controllerMaarten/FromActuators/RA/ToMotorAngle_rad/MotorAngle ==
  data: pos input; gearboxRatio parameter; encoderCounts_rev parameter; pos_mot_rad output; JointAngle_rad input; SpringDeflection_rad input; Calibrate input
function pos_mot_rad  = ...
    PosActValDecode(pos, gearboxRatio, encoderCounts_rev, JointAngle_rad, SpringDeflection_rad, Calibrate)
%#codegen
%
% The output is the motor angle, converted to AFTER the gearbox
% (thus the value you get here is equal to the true rotor angle divided by
% the gearbox ratio). It has the same order of magnitude, and is directly
% comparable to the joint angle and spring angle.

% This block includes calibration such that (ideally) the motor angle is
% zero when the joint angle and spring deflection are zero as well. Before
% the calibration has occurred, the output of this function is -10*. This
% is chosen such that the value is always outside the allowed motor angle
% range; this prevents the drive from being allowed to turn on (since we
% have no multiple-rotation parts, we can never have a value larger than
% -2pi. Chose -10 because it is not ridiculously large so the vertical
% scaling of graphs will not be affected that severely.
% 
%
% * I wanted to use -inf as starting function, but I'm not sure whether
%   that will be handled correctly in all cases.

persistent isCalibrated;
persistent offset;

if isempty(isCalibrated)
    isCalibrated = 0;
    offset = 0;
end

pos_inc = double(pos);

if Calibrate
    pos_mot_rad_temp = pos_inc * 2*pi / (encoderCounts_rev * gearboxRatio); % The angle we read from the motor encoder
    target_pos_mot_rad = JointAngle_rad + SpringDeflection_rad; % This is what we should read
    offset = target_pos_mot_rad - pos_mot_rad_temp;
    isCalibrated = 1;
end

if isCalibrated
    pos_mot_rad = pos_inc * 2*pi / (encoderCounts_rev * gearboxRatio) + offset;
else
    pos_mot_rad = -10;
end

== matlab function WEankle_controllerMaarten/Ankle Controller/MATLAB Function7 ==
  data: e0 input; G input; SolGains output; COMd input
function SolGains  = CombineSoleusGains(e0,G,COMd)
% input arguments:

SolGains = [e0; G; COMd];
